simulink model "EEE411L_exp_02_Matlab_2024b"  (R2024b)
settings: Solver=VariableStepAuto  StartTime=0.0  StopTime=10.0  RelTol=1e-3
settings Model: Creator=fahim  LastModifiedBy=fahim
settings ConfigComp: CovBoundaryAbsTol=1.0e-5

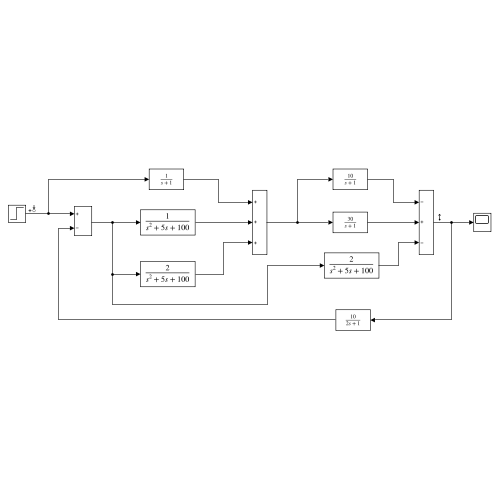
[thumbnail: Simulink's stored preview of the top-level diagram]
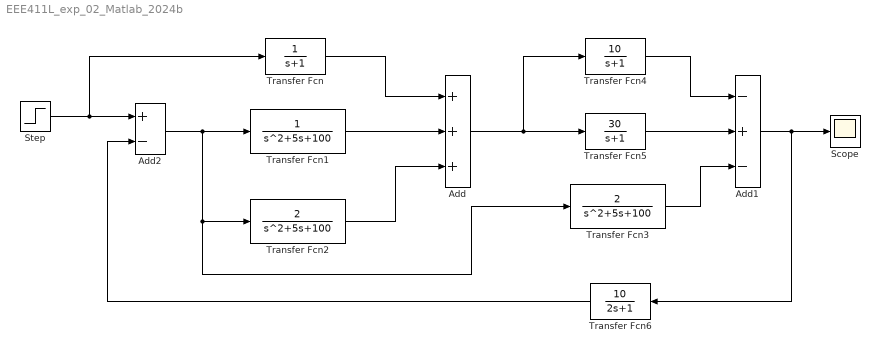
== system EEE411L_exp_02_Matlab_2024b ==
  Add : Sum  Inputs=+++
  Add1 : Sum  Inputs=-+-
  Add2 : Sum  Inputs=+-
  Scope : Scope
  Step : Step  Time=0  SampleTime=0
  Transfer Fcn : TransferFcn  Denominator=[1 1]
  Transfer Fcn1 : TransferFcn  Denominator=[1 5 100]
  Transfer Fcn2 : TransferFcn  Numerator=[2]  Denominator=[1 5 100]
  Transfer Fcn3 : TransferFcn  Numerator=[2]  Denominator=[1 5 100]
  Transfer Fcn4 : TransferFcn  Numerator=[10]  Denominator=[1 1]
  Transfer Fcn5 : TransferFcn  Numerator=[30]  Denominator=[1 1]
  Transfer Fcn6 : TransferFcn  Numerator=[10]  Denominator=[2 1]
  wires:
  Transfer Fcn/1 -> Add/1
  Transfer Fcn1/1 -> Add/2
  Transfer Fcn2/1 -> Add/3
  Add/1 -> Transfer Fcn4/1, Transfer Fcn5/1
  Transfer Fcn5/1 -> Add1/2
  Transfer Fcn4/1 -> Add1/1
  Transfer Fcn3/1 -> Add1/3
  Add2/1 -> Transfer Fcn2/1, Transfer Fcn3/1, Transfer Fcn1/1
  Transfer Fcn6/1 -> Add2/2
  Add1/1 -> Scope/1, Transfer Fcn6/1
  Step/1 -> Transfer Fcn/1, Add2/1
